simulink model "Controller0"  (R2020b)
settings: Solver=FixedStepDiscrete  StartTime=0.0  StopTime=3  FixedStep=1e-06  RelTol=1e-3
settings Model: ExtModeTrigDuration=2  Creator=拾夕  LastModifiedBy=拾夕
settings DataIOCC: SaveOutput=off  SaveTime=off
settings OptimizationCC: EnhancedBackFolding=on  PassReuseOutputArgsAs=Individual arguments  MaxStackSize=64  OptimizeBlockOrder=speed  DifferentSizesBufferReuse=on  OptimizationCustomize=off  EfficientTunableParamExpr=on
settings DebuggingCC: ParameterTunabilityLossMsg=error
settings HardwareCC: ProdBitPerInt=16  ProdBitPerPointer=16  ProdBitPerSizeT=16  ProdBitPerPtrDiffT=16  ProdLargestAtomicFloat=None  ProdWordSize=8  ProdHWDeviceType=Atmel->AVR
settings SFSimCC: MATLABDynamicMemAlloc=off
settings RTWCC: Description=Embedded Coder  SystemTargetFile=ert.tlc  HardwareBoard=Arduino Uno  GenCodeOnly=on  TemplateMakefile=ert_default_tmf  GenerateReport=on  RetainRTWFile=on  Toolchain=Arduino AVR  BuildConfiguration=Faster Runs  LaunchReport=on  GenerateWebview=on  GenerateCodeMetricsReport=on
settings CodeAppCC: ForceParamTrailComments=on  IgnoreCustomStorageClasses=off  OperatorAnnotations=on  SimulinkDataObjDesc=on  SFDataObjDesc=on  InsertBlockDesc=on
settings ERTTargetCC: CodeInterfacePackaging=Reusable function  SupportContinuousTime=on  SupportVariableSizeSignals=on  ExtModeStaticAllocSize=250

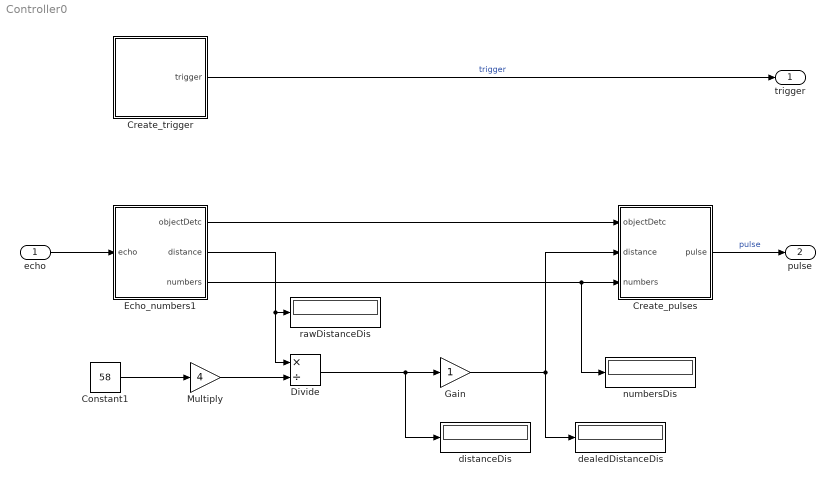
== system Controller0 ==
  echo : Inport  OutDataTypeStr=single  PortDimensions=1  SampleTime=[9.9999999999999995e-07,0]
  Constant1 : Constant  Value=58
  Create_pulses : Stateflow chart  TreatAsAtomicUnit=on
  Create_trigger : Stateflow chart  TreatAsAtomicUnit=on
  Divide : Product  Inputs=*/  OutDataTypeStr=single
  Echo_numbers1 : Stateflow chart  TreatAsAtomicUnit=on
  Gain : Gain  OutDataTypeStr=int16  RndMeth=Nearest
  Multiply : Gain  Gain=4
  dealedDistanceDis : Display
  distanceDis : Display
  numbersDis : Display
  rawDistanceDis : Display
  trigger : Outport  OutDataTypeStr=single  PortDimensions=1  SampleTime=[9.9999999999999995e-07,0]
  pulse : Outport  Port=2  OutDataTypeStr=single  PortDimensions=1  SampleTime=[9.9999999999999995e-07,0]
  wires:
  Echo_numbers1/2(distance) -> Divide/1, rawDistanceDis/1
  Echo_numbers1/1(objectDetc) -> Create_pulses/1(objectDetc)
  Constant1/1 -> Multiply/1
  Create_pulses/1(pulse) -> pulse/1  "pulse"
  Multiply/1 -> Divide/2
  echo/1 -> Echo_numbers1/1(echo)
  Divide/1 -> distanceDis/1, Gain/1
  Create_trigger/1(trigger) -> trigger/1  "trigger"
  Gain/1 -> dealedDistanceDis/1, Create_pulses/2(distance)
  Echo_numbers1/3(numbers) -> numbersDis/1, Create_pulses/3(numbers)

== stateflow chart Controller0/Create_trigger ==
  state TriggerOff
    en:
    trigger=0;
  state TriggerOn
    en:
    trigger=1;
  (default) -> TriggerOff
  TriggerOff -> TriggerOn : after(60,msec)
  TriggerOn -> TriggerOff : after(20,usec)
  data: trigger output single

== stateflow chart Controller0/Create_pulses ==
  state Medile
  state SignalOne
    en:
    pulse=1;
  state SignalZero
    en:
    pulse=0;
  (default) -> Medile
  Medile -> SignalOne [order 2] : after(500,msec)
  Medile -> SignalOne [order 1] : [numbers>=4]
  (junction 9) -> (junction 11) [order 1] : [objectDetc==0]
  SignalOne -> (junction 9)
  (junction 35) -> SignalOne : after(100-distance,msec)
  (junction 11) -> SignalZero : after(0.5,sec)
  (junction 9) -> (junction 13) [order 2] : [objectDetc==1]
  (junction 26) -> SignalOne : after(0.5,sec)
  (junction 32) -> SignalOne : after(0.25,sec)
  (junction 13) -> (junction 15) [order 1] : [distance>=10&&distance<=100]
  (junction 13) -> (junction 18) [order 2] : [distance<10||distance>100]
  (junction 15) -> SignalZero : after(distance,msec)
  (junction 30) -> (junction 35) [order 2] : [distance>=10&&distance<=100]
  SignalZero -> (junction 26) [order 1] : [objectDetc==0]
  (junction 18) -> SignalZero : after(0.25,sec)
  SignalZero -> (junction 30) [order 2] : [objectDetc==1]
  (junction 30) -> (junction 32) [order 1] : [distance<10||distance>100]
  data: objectDetc input single; distance input int16; pulse output single; numbers input single

== stateflow chart Controller0/Echo_numbers1 ==
  settings: updateMethod=DISCRETE  sampleTime=0.000001
  state CountNums
    du:
    distance = distance + 1;
  state Init
    en:
    objectDetc=0;
    distance=0;
    numbers=0;
  state Wait
  state Stop
    en:
    objectDetc=1;
    numbers = numbers + 1;
  Wait -> CountNums : [echo==1]
  CountNums -> Stop : [echo==0]
  (default) -> Init
  Init -> Wait
  Stop -> Wait : [numbers<4]
  data: objectDetc output single; distance output single; echo input single; numbers output single
